simulink model "Servo_Control"  (R2018b)
settings: Solver=VariableStepAuto  StartTime=0.0  StopTime=10.0  RelTol=1e-3
values from neighbouring files (symbols this model uses):
  A = zeros(5,5)    [kalmanfilter.m]    (also in model_2017.m = [[0  0   0   0                0             0   1           ; model_rough.m; model_v2.m = [[0  0   0   0                0             0   1           ; model_v3.m = [[   0   0                     0   0           0           1)
  B = zeros(5,6)    [kalmanfilter.m]    (also in model_2017.m = [[0      0      0      0     ];                        [0   ; model_rough.m; model_v2.m = [[0      0      0      0     ];                        [0   ; model_v3.m = [[0      0      0      0      0      0             ];       )
  C = eye(5)    [kalmanfilter.m]    (also in model_2017.m = [[0  0   0   0   0   0   1   0   0   0   0   0]; model_rough.m; model_v2.m = [[0  0   0   0   0   0   1   0   0   0   0   0]; model_v3.m = [[0   0   0   1   0   0   0   0])
  K = []    [kalmanfilter.m]    (also in model_rough.m = place(A, B, polevec); model_v3.m = Kaug(1:8))
  Ka = Kaug(9:14)    [model_v3.m]
settings Model: Creator=Rishabh  LastModifiedBy=Rishabh

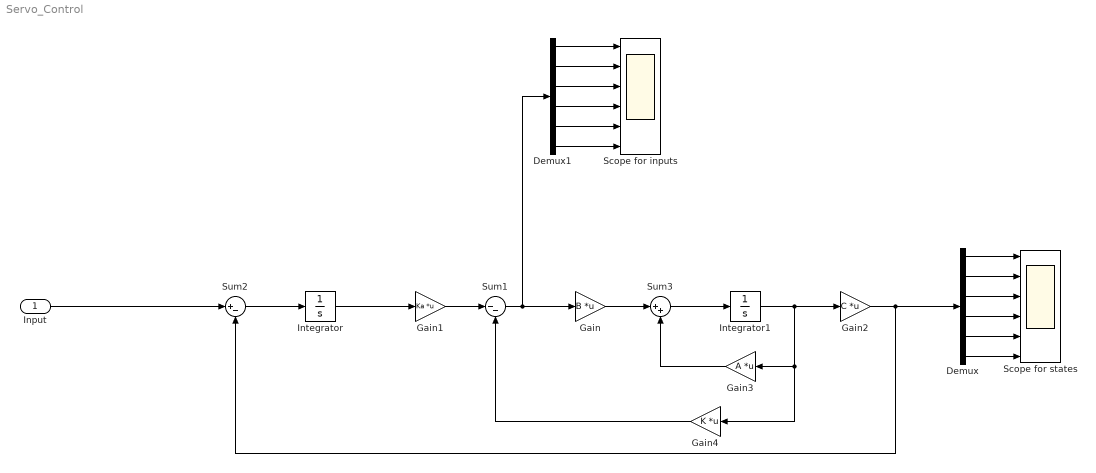
== system Servo_Control ==
  Input : Inport
  Demux : Demux  Outputs=6
  Demux1 : Demux  Outputs=6
  Gain : Gain  Gain=B  Multiplication=Matrix(K*u)
  Gain1 : Gain  Gain=Ka  Multiplication=Matrix(K*u)
  Gain2 : Gain  Gain=C  Multiplication=Matrix(K*u)
  Gain3 : Gain  Gain=A  Multiplication=Matrix(K*u)
  Gain4 : Gain  Gain=K  Multiplication=Matrix(K*u)
  Integrator : Integrator
  Integrator1 : Integrator
  Scope for inputs : Scope  NumInputPorts=6
  Scope for states : Scope  NumInputPorts=6
  Sum1 : Sum  Inputs=|--
  Sum2 : Sum  Inputs=|+-
  Sum3 : Sum  Inputs=|++
  wires:
  Input/1 -> Sum2/1
  Integrator/1 -> Gain1/1
  Sum2/1 -> Integrator/1
  Gain1/1 -> Sum1/1
  Sum1/1 -> Demux1/1, Gain/1
  Gain/1 -> Sum3/1
  Sum3/1 -> Integrator1/1
  Integrator1/1 -> Gain4/1, Gain3/1, Gain2/1
  Gain2/1 -> Sum2/2, Demux/1
  Demux/1 -> Scope for states/1
  Demux/2 -> Scope for states/2
  Demux/3 -> Scope for states/3
  Demux/4 -> Scope for states/4
  Demux/5 -> Scope for states/5
  Demux/6 -> Scope for states/6
  Gain3/1 -> Sum3/2
  Gain4/1 -> Sum1/2
  Demux1/1 -> Scope for inputs/1
  Demux1/2 -> Scope for inputs/2
  Demux1/3 -> Scope for inputs/3
  Demux1/4 -> Scope for inputs/4
  Demux1/5 -> Scope for inputs/5
  Demux1/6 -> Scope for inputs/6
